simulink model "Vibrations"  (R2026a)
settings: Solver=VariableStepAuto  StopTime=5
settings Model: Creator=thabi  LastModifiedBy=thabi

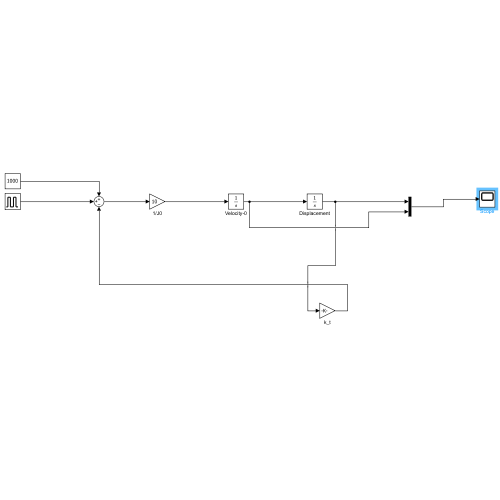
[thumbnail: Simulink's stored preview of the top-level diagram]
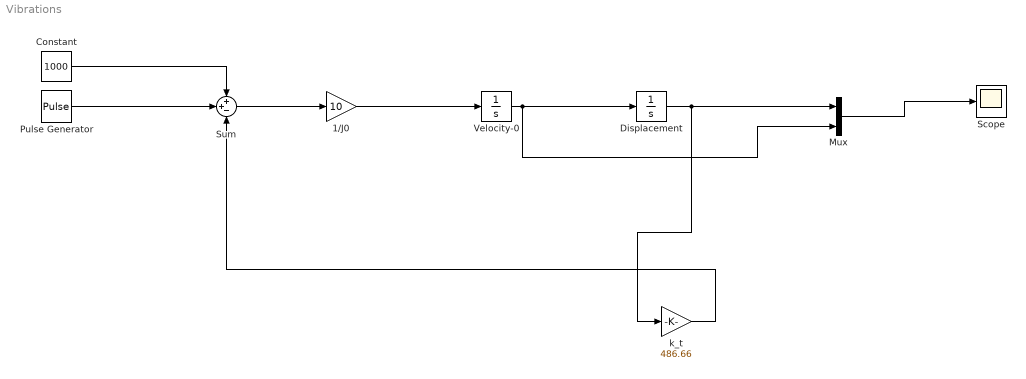
== system Vibrations ==
  1/J0 : Gain  Gain=10
  Constant : Constant  Value=1000  VectorParams1D=off
  Displacement : Integrator  ZeroCross=off
  Mux : Mux  Inputs=2
  Pulse Generator : DiscretePulseGenerator  PulseType=Time based  Amplitude=100  Period=0.00375  PulseWidth=5  VectorParams1D=off
  Scope : Scope
      settings: ActiveDisplayYMinimum=-180.1853427594811  ActiveDisplayYMaximum=180.18568780086898  DataLoggingVariableName=simout
  Sum : Sum  Inputs=++-
  Velocity-0 : Integrator  ZeroCross=off
  k_t : Gain  Gain=486.66
  wires:
  Constant/1 -> Sum/1
  Pulse Generator/1 -> Sum/2
  Sum/1 -> 1/J0/1
  1/J0/1 -> Velocity-0/1
  Velocity-0/1 -> Mux/2, Displacement/1
  Displacement/1 -> k_t/1, Mux/1
  Mux/1 -> Scope/1
  k_t/1 -> Sum/3
